simulink subsystem "AeroPropRefFranc"  (R2024b)
settings: Solver=VariableStepAuto  StartTime=0.0  StopTime=10.0  RelTol=1e-3
undefined symbols (not defined in the file or in its folder): ess, Force_b, Fprop_r, geom, H_b, Hdot_b, Moment_b, mot, mot2, mot3, mot4, Mprop_r, propel, propel2, propel3, propel4, pxf_diagram_options, SimIn, SimPar, tc, tc2, tc3, tc4
libraries: simulink x8, slpidlib x4, starslibAxisTransformations x2, libAxisTransformations x2
(part 7 of 10)

== system AeroPropRefFranc/Propulsion and Aerodynamic Forces and Moments/S-Function/Battery Model/powerplant/mot2/ctrl/dmd/parameter_selection ==
  inport-main_info_bus-1 : Inport
  select_main_info_bus : BusSelector  OutputSignals=apc_info_bus.apc_ctrl_dt2_simu,env_info_bus.env_plant_density_simu,apa_info_bus.powerplant_info_bus.ess.ctrl.ess_ctrl_pwr_max_pro_simu,apa_info_bus.powerplant_info_bus.propel2.propel2_plant_speed_simu,apa_info_bus.powerplant_info_bus.tc2.tc2_plant_spd_in_simu
  outport-apc_ctrl_dt2_simu-1 : Outport
  outport-env_plant_density_simu-2 : Outport  Port=2
  outport-ess_ctrl_pwr_max_pro_simu-3 : Outport  Port=3
  outport-propel2_plant_speed_simu-4 : Outport  Port=4
  outport-tc2_plant_spd_in_simu-5 : Outport  Port=5
  wires:
  select_main_info_bus/5 -> outport-tc2_plant_spd_in_simu-5/1  "<tc2_plant_spd_in_simu>"
  select_main_info_bus/4 -> outport-propel2_plant_speed_simu-4/1  "<propel2_plant_speed_simu>"
  select_main_info_bus/3 -> outport-ess_ctrl_pwr_max_pro_simu-3/1  "<ess_ctrl_pwr_max_pro_simu>"
  select_main_info_bus/2 -> outport-env_plant_density_simu-2/1  "<env_plant_density_simu>"
  select_main_info_bus/1 -> outport-apc_ctrl_dt2_simu-1/1  "<apc_ctrl_dt2_simu>"
  inport-main_info_bus-1/1 -> select_main_info_bus/1

== system AeroPropRefFranc/Propulsion and Aerodynamic Forces and Moments/S-Function/Battery Model/powerplant/mot2/plant/mot2_plant_map_Pelec_funTW_volt_in/electric machine filter ==
  trq : Inport
  Interval Test : simulink/Logic and Bit Operations/Interval Test  IntervalClosedRight=on  uplimit=0.02  IntervalClosedLeft=on  lowlimit=-0.02  OutDataTypeStr=boolean
  Switch : Switch  Threshold=0.5  SaturateOnIntegerOverflow=off  InputSameDT=off
  electric machine time response : TransferFcn  Denominator=[mot2.plant.init.time_response 1]
  filtered : Outport
  wires:
  electric machine time response/1 -> Switch/3
  Interval Test/1 -> Switch/2
  trq/1 -> Switch/1, Interval Test/1, electric machine time response/1
  Switch/1 -> filtered/1

== system AeroPropRefFranc/Propulsion and Aerodynamic Forces and Moments/S-Function/Battery Model/powerplant/mot2/plant/mot2_plant_map_Pelec_funTW_volt_in/max torque  ==
  cmd : Inport
  speed : Inport  Port=2
  torque : Inport  Port=3
  Abs : Abs
  Cont trq max - Prop : Subsystem  mask{x=mot2.plant.init.trq_pos_cont.idx1_spd, map=mot2.plant.init.trq_pos_cont.map}
      mask Display: image(imread('map1D.jpg','jpeg'))
  Cont trq max - Regen : Subsystem  mask{x=mot2.plant.init.trq_neg_cont.idx1_spd, map=mot2.plant.init.trq_neg_cont.map}
      mask Display: image(imread('map1D.jpg','jpeg'))
  Heat index : Subsystem
  Memory : Memory
  Peak trq max - Prop : Subsystem  mask{x=mot2.plant.init.trq_pos_max.idx1_spd, map=mot2.plant.init.trq_pos_max.map}
      mask Display: image(imread('map1D.jpg','jpeg'))
  Peak trq max - Regen : Subsystem  mask{x=mot2.plant.init.trq_neg_max.idx1_spd, map=mot2.plant.init.trq_neg_max.map}
      mask Display: image(imread('map1D.jpg','jpeg'))
  Product2 : Product  InputSameDT=on  SaturateOnIntegerOverflow=on  OutDataTypeStr=Inherit: Same as first input
  Product3 : Product  InputSameDT=on  SaturateOnIntegerOverflow=on  OutDataTypeStr=Inherit: Same as first input
  Product5 : Product  InputSameDT=on  SaturateOnIntegerOverflow=on  OutDataTypeStr=Inherit: Same as first input
  Sign : Signum
  Sum : Sum  InputSameDT=on  SaturateOnIntegerOverflow=on  OutDataTypeStr=Inherit: Same as first input
  Sum1 : Sum  Inputs=-+  InputSameDT=on  SaturateOnIntegerOverflow=on  OutDataTypeStr=Inherit: Same as first input
  Switch : Switch  InputSameDT=off
  Switch1 : Switch  InputSameDT=off
  cst : Constant
  max torque : Outport
  heat index : Outport  Port=2
  wires:
  Heat index/1(Heat index) -> heat index/1, Sum1/1, Product2/2
  cst/1 -> Sum1/2
  Product3/1 -> Sum/2
  Sum1/1 -> Product3/1
  Product2/1 -> Sum/1
  Switch1/1 -> Product3/2
  Switch/1 -> Heat index/1(cont torque), Product2/1
  Peak trq max - Regen/1(output) -> Switch1/3
  Peak trq max - Prop/1(output) -> Switch1/1
  Cont trq max - Regen/1(output) -> Switch/3
  Cont trq max - Prop/1(output) -> Switch/1
  speed/1 -> Memory/1
  cmd/1 -> Switch/2, Switch1/2
  torque/1 -> Heat index/2(torque)
  Abs/1 -> Product5/2
  Sum/1 -> Abs/1, Sign/1
  Product5/1 -> max torque/1
  Sign/1 -> Product5/1
  Memory/1 -> Peak trq max - Prop/1(input x), Peak trq max - Regen/1(input x), Cont trq max - Regen/1(input x), Cont trq max - Prop/1(input x)

== system AeroPropRefFranc/Propulsion and Aerodynamic Forces and Moments/S-Function/Battery Model/powerplant/mot2/plant/mot2_plant_map_Pelec_funTW_volt_in/non-zero division ==
  note: original idea from Phil Sharer - ANL
      | original formula: u[1]\(u[2]+eps)*(u[2]!=0)
      | changes done by Gerald ZINI (dgey) - ANL (05\02\2001)
  note: (u[2]==0) is true then returns 1, thus (u[2]+(u[2]==0)) is equal to 0+1=1
  note: if u[2] == 0, then output == 0:
  note: (u[2]!=0) is false then returns 0
  note: and finally, the expression is: (u[1] \ 1) * 0 = 0
  note: (u[2]==0) is false then returns 0, thus (u[2]+(u[2]==0)) is equal to u[2]+0=u[2]
  note: if u[2] != 0, then output == u[1]\u[2]:
  note: (u[2]!=0) is true then returns 1
  note: and finally, the expression is: (u[1] \ u[2]) * 1 = u[1] \ u[2]
  In1 : Inport
  In2 : Inport  Port=2
  Fcn : Fcn  Expr=u[1]/(u[2]+(u[2]==0))*(u[2]!=0)
  Mux : Mux  Inputs=2
  Out1 : Outport
  wires:
  Mux/1 -> Fcn/1
  In1/1 -> Mux/1
  Fcn/1 -> Out1/1
  In2/1 -> Mux/2

== system AeroPropRefFranc/Propulsion and Aerodynamic Forces and Moments/S-Function/Battery Model/powerplant/mot3/ctrl/cmd/mot3_ctrl_cmd_map_Pelec_funTW_volt_in ==
  mot_plant_spd_out_simu : Inport
  mot_ctrl_trs_trq_simu : Inport  Port=2
  mot_ctrl_cstr_trq_max_pos_simu : Inport  Port=3
  mot_ctrl_cstr_trq_max_neg_simu : Inport  Port=4
  Abs : Abs
  Abs1 : Abs
  Abs2 : Abs
  Fcn : Fcn  Expr=(u>=0) - (u<0)
  Product : Product  SaturateOnIntegerOverflow=on  OutDataTypeStr=Inherit: Same as first input
  Product1 : Product  SaturateOnIntegerOverflow=on  OutDataTypeStr=Inherit: Same as first input
  Subsystem2 : Subsystem
      mask Display: disp('divider')
  Switch : Switch  InputSameDT=off
  "[-1, 1]" : Saturate  UpperLimit=1  LowerLimit=-1
  avoid zero output : Subsystem
  mot_ctrl_cmd_simu : Outport
  wires:
  Fcn/1 -> Product1/1
  "[-1, 1]"/1 -> Product1/2
  Abs2/1 -> Switch/3
  Abs1/1 -> Switch/1
  Abs/1 -> Subsystem2/1(In1)
  mot_ctrl_trs_trq_simu/1 -> Abs/1, Product/1
  Subsystem2/1(Out1) -> "[-1, 1]"/1
  Switch/1 -> Subsystem2/2(In2)
  Product/1 -> Fcn/1, Switch/2
  mot_plant_spd_out_simu/1 -> avoid zero output/1(In1)
  mot_ctrl_cstr_trq_max_neg_simu/1 -> Abs2/1
  mot_ctrl_cstr_trq_max_pos_simu/1 -> Abs1/1
  Product1/1 -> [mot3_ctrl_cmd_simu]
  [mot3_ctrl_cmd_simu] -> mot_ctrl_cmd_simu/1  "mot_ctrl_cmd_simu"
  avoid zero output/1(Out1) -> Product/2

== system AeroPropRefFranc/Propulsion and Aerodynamic Forces and Moments/S-Function/Battery Model/powerplant/mot3/ctrl/cmd/parameter_out ==
  inport-mot3_ctrl_cmd_simu : Inport
  Toworkspace-mot3_ctrl_cmd_simu : ToWorkspace  VariableName=mot3_ctrl_cmd_simu  SampleTime=pxf_diagram_options.workspace_sample_time
      settings: Decimation=pxf_diagram_options.decimation
  create_system_info_bus : BusCreator  Inputs=1
  outport-system_info_bus : Outport
  wires:
  inport-mot3_ctrl_cmd_simu/1 -> Toworkspace-mot3_ctrl_cmd_simu/1, create_system_info_bus/1  "mot3_ctrl_cmd_simu"
  create_system_info_bus/1 -> outport-system_info_bus/1

== system AeroPropRefFranc/Propulsion and Aerodynamic Forces and Moments/S-Function/Battery Model/powerplant/mot3/ctrl/cmd/parameter_selection ==
  inport-main_info_bus-1 : Inport
  select_main_info_bus : BusSelector  OutputSignals=apa_info_bus.powerplant_info_bus.mot3.plant.mot3_plant_spd_out_simu,apa_info_bus.powerplant_info_bus.mot3.ctrl.dmd.mot3_ctrl_trs_trq_simu,apa_info_bus.powerplant_info_bus.mot3.ctrl.cstr.mot3_ctrl_cstr_trq_max_pos_simu,apa_info_bus.powerplant_info_bus.mot3.ctrl.cstr.mot3_ctrl_cstr_trq_max_neg_simu
  outport-mot3_plant_spd_out_simu-1 : Outport
  outport-mot3_ctrl_trs_trq_simu-2 : Outport  Port=2
  outport-mot3_ctrl_cstr_trq_max_pos_simu-3 : Outport  Port=3
  outport-mot3_ctrl_cstr_trq_max_neg_simu-4 : Outport  Port=4
  wires:
  select_main_info_bus/4 -> outport-mot3_ctrl_cstr_trq_max_neg_simu-4/1  "<mot3_ctrl_cstr_trq_max_neg_simu>"
  select_main_info_bus/3 -> outport-mot3_ctrl_cstr_trq_max_pos_simu-3/1  "<mot3_ctrl_cstr_trq_max_pos_simu>"
  select_main_info_bus/2 -> outport-mot3_ctrl_trs_trq_simu-2/1  "<mot3_ctrl_trs_trq_simu>"
  select_main_info_bus/1 -> outport-mot3_plant_spd_out_simu-1/1  "<mot3_plant_spd_out_simu>"
  inport-main_info_bus-1/1 -> select_main_info_bus/1

== system AeroPropRefFranc/Propulsion and Aerodynamic Forces and Moments/S-Function/Battery Model/powerplant/mot3/ctrl/cstr/mot3_ctrl_cstr_map_Pelec_funTW_volt_in ==
  mot_plant_spd_out_simu : Inport
  mot_plant_temp_coeff_simu : Inport  Port=2
  Continuous torque - Prop : Subsystem  mask{x=mot3.plant.init.trq_pos_cont.idx1_spd, map=mot3.plant.init.trq_pos_cont.map}
      mask Display: image(imread('map1D.jpg','jpeg'))
  Continuous torque _regen : Subsystem  mask{x=mot3.plant.init.trq_neg_cont.idx1_spd, map=mot3.plant.init.trq_neg_cont.map}
      mask Display: image(imread('map1D.jpg','jpeg'))
  Mux1 : Mux  Inputs=3
  Mux2 : Mux  Inputs=3
  Peak torque - Prop : Subsystem  mask{x=mot3.plant.init.trq_pos_max.idx1_spd, map=mot3.plant.init.trq_pos_max.map}
      mask Display: image(imread('map1D.jpg','jpeg'))
  Peak torque _regen : Subsystem  mask{x=mot3.plant.init.trq_neg_max.idx1_spd, map=mot3.plant.init.trq_neg_max.map}
      mask Display: image(imread('map1D.jpg','jpeg'))
  Torque1 : Fcn  Expr=u[3]*(u[2] - u[1]) + u[1]
  max torque available from meca side : Fcn  Expr=u[3]*(u[2] - u[1]) + u[1]
  mot_ctrl_cstr_trq_pk_pos_simu : Outport
  mot_ctrl_cstr_trq_max_pos_simu : Outport  Port=2
  mot_ctrl_cstr_trq_pk_neg_simu : Outport  Port=3
  mot_ctrl_cstr_trq_max_neg_simu : Outport  Port=4
  mot_ctrl_cstr_trq_cont_pos_simu : Outport  Port=5
  mot_ctrl_cstr_trq_cont_neg_simu : Outport  Port=6
  mot_ctrl_cstr_temp_coeff_simu : Outport  Port=7
  wires:
  max torque available from meca side/1 -> [mot3_ctrl_cstr_trq_max_pos_simu]
  Torque1/1 -> [mot3_ctrl_cstr_trq_max_neg_simu]
  Continuous torque - Prop/1(output) -> Mux2/2, [mot3_ctrl_cstr_trq_cont_pos_simu]
  Mux2/1 -> max torque available from meca side/1
  Continuous torque _regen/1(output) -> Mux1/2, [mot3_ctrl_cstr_trq_cont_neg_simu]
  Mux1/1 -> Torque1/1
  mot_plant_temp_coeff_simu/1 -> Mux1/3, Mux2/3, [mot3_ctrl_cstr_temp_coeff_simu]
  Peak torque - Prop/1(output) -> Mux2/1, [mot3_ctrl_cstr_trq_pk_pos_simu]
  Peak torque _regen/1(output) -> [mot3_ctrl_cstr_trq_pk_neg_simu], Mux1/1
  mot_plant_spd_out_simu/1 -> Continuous torque - Prop/1(input x), Peak torque _regen/1(input x), Continuous torque _regen/1(input x), Peak torque - Prop/1(input x)
  [mot3_ctrl_cstr_trq_pk_pos_simu] -> mot_ctrl_cstr_trq_pk_pos_simu/1  "mot_ctrl_cstr_trq_pk_pos_simu"
  [mot3_ctrl_cstr_trq_max_pos_simu] -> mot_ctrl_cstr_trq_max_pos_simu/1  "mot_ctrl_cstr_trq_max_pos_simu"
  [mot3_ctrl_cstr_trq_max_neg_simu] -> mot_ctrl_cstr_trq_max_neg_simu/1  "mot_ctrl_cstr_trq_max_neg_simu"
  [mot3_ctrl_cstr_trq_pk_neg_simu] -> mot_ctrl_cstr_trq_pk_neg_simu/1  "mot_ctrl_cstr_trq_pk_neg_simu"
  [mot3_ctrl_cstr_trq_cont_pos_simu] -> mot_ctrl_cstr_trq_cont_pos_simu/1  "mot_ctrl_cstr_trq_cont_pos_simu"
  [mot3_ctrl_cstr_trq_cont_neg_simu] -> mot_ctrl_cstr_trq_cont_neg_simu/1  "mot_ctrl_cstr_trq_cont_neg_simu"
  [mot3_ctrl_cstr_temp_coeff_simu] -> mot_ctrl_cstr_temp_coeff_simu/1  "mot_ctrl_cstr_temp_coeff_simu"

== system AeroPropRefFranc/Propulsion and Aerodynamic Forces and Moments/S-Function/Battery Model/powerplant/mot3/ctrl/cstr/parameter_out ==
  inport-mot3_ctrl_cstr_trq_pk_pos_simu : Inport
  inport-mot3_ctrl_cstr_trq_max_pos_simu : Inport  Port=2
  inport-mot3_ctrl_cstr_trq_pk_neg_simu : Inport  Port=3
  inport-mot3_ctrl_cstr_trq_max_neg_simu : Inport  Port=4
  inport-mot3_ctrl_cstr_trq_cont_pos_simu : Inport  Port=5
  inport-mot3_ctrl_cstr_trq_cont_neg_simu : Inport  Port=6
  inport-mot3_ctrl_cstr_temp_coeff_simu : Inport  Port=7
  Ground_1 : Ground
  Toworkspace-mot3_ctrl_cstr_temp_coeff_simu : ToWorkspace  VariableName=mot3_ctrl_cstr_temp_coeff_simu  SampleTime=pxf_diagram_options.workspace_sample_time
      settings: Decimation=pxf_diagram_options.decimation
  Toworkspace-mot3_ctrl_cstr_trq_cont_neg_simu : ToWorkspace  VariableName=mot3_ctrl_cstr_trq_cont_neg_simu  SampleTime=pxf_diagram_options.workspace_sample_time
      settings: Decimation=pxf_diagram_options.decimation
  Toworkspace-mot3_ctrl_cstr_trq_cont_pos_simu : ToWorkspace  VariableName=mot3_ctrl_cstr_trq_cont_pos_simu  SampleTime=pxf_diagram_options.workspace_sample_time
      settings: Decimation=pxf_diagram_options.decimation
  Toworkspace-mot3_ctrl_cstr_trq_max_neg_simu : ToWorkspace  VariableName=mot3_ctrl_cstr_trq_max_neg_simu  SampleTime=pxf_diagram_options.workspace_sample_time
      settings: Decimation=pxf_diagram_options.decimation
  Toworkspace-mot3_ctrl_cstr_trq_max_pos_simu : ToWorkspace  VariableName=mot3_ctrl_cstr_trq_max_pos_simu  SampleTime=pxf_diagram_options.workspace_sample_time
      settings: Decimation=pxf_diagram_options.decimation
  Toworkspace-mot3_ctrl_cstr_trq_pk_neg_simu : ToWorkspace  VariableName=mot3_ctrl_cstr_trq_pk_neg_simu  SampleTime=pxf_diagram_options.workspace_sample_time
      settings: Decimation=pxf_diagram_options.decimation
  Toworkspace-mot3_ctrl_cstr_trq_pk_pos_simu : ToWorkspace  VariableName=mot3_ctrl_cstr_trq_pk_pos_simu  SampleTime=pxf_diagram_options.workspace_sample_time
      settings: Decimation=pxf_diagram_options.decimation
  create_system_info_bus : BusCreator  Inputs=2
  outport-system_info_bus : Outport
  outport-cstr_bus : Outport  Port=2
  wires:
  Ground_1/1 -> outport-cstr_bus/1
  inport-mot3_ctrl_cstr_temp_coeff_simu/1 -> Toworkspace-mot3_ctrl_cstr_temp_coeff_simu/1
  inport-mot3_ctrl_cstr_trq_cont_neg_simu/1 -> Toworkspace-mot3_ctrl_cstr_trq_cont_neg_simu/1
  inport-mot3_ctrl_cstr_trq_cont_pos_simu/1 -> Toworkspace-mot3_ctrl_cstr_trq_cont_pos_simu/1
  inport-mot3_ctrl_cstr_trq_max_neg_simu/1 -> Toworkspace-mot3_ctrl_cstr_trq_max_neg_simu/1, create_system_info_bus/2  "mot3_ctrl_cstr_trq_max_neg_simu"
  inport-mot3_ctrl_cstr_trq_pk_neg_simu/1 -> Toworkspace-mot3_ctrl_cstr_trq_pk_neg_simu/1
  inport-mot3_ctrl_cstr_trq_max_pos_simu/1 -> Toworkspace-mot3_ctrl_cstr_trq_max_pos_simu/1, create_system_info_bus/1  "mot3_ctrl_cstr_trq_max_pos_simu"
  inport-mot3_ctrl_cstr_trq_pk_pos_simu/1 -> Toworkspace-mot3_ctrl_cstr_trq_pk_pos_simu/1
  create_system_info_bus/1 -> outport-system_info_bus/1

== system AeroPropRefFranc/Propulsion and Aerodynamic Forces and Moments/S-Function/Battery Model/powerplant/mot3/ctrl/cstr/parameter_selection ==
  inport-main_info_bus-1 : Inport
  select_main_info_bus : BusSelector  OutputSignals=apa_info_bus.powerplant_info_bus.mot3.plant.mot3_plant_spd_out_simu,apa_info_bus.powerplant_info_bus.mot3.plant.mot3_plant_temp_coeff_simu
  outport-mot3_plant_spd_out_simu-1 : Outport
  outport-mot3_plant_temp_coeff_simu-2 : Outport  Port=2
  wires:
  select_main_info_bus/2 -> outport-mot3_plant_temp_coeff_simu-2/1  "<mot3_plant_temp_coeff_simu>"
  select_main_info_bus/1 -> outport-mot3_plant_spd_out_simu-1/1  "<mot3_plant_spd_out_simu>"
  inport-main_info_bus-1/1 -> select_main_info_bus/1

== system AeroPropRefFranc/Propulsion and Aerodynamic Forces and Moments/S-Function/Battery Model/powerplant/mot3/ctrl/dmd/mot3_ctrl_dmd_uas ==
  apc_ctrl_dt_simu : Inport
  env_plant_density_simu : Inport  Port=2
  ess_ctrl_pwr_max_pro_simu : Inport  Port=3
  propel_plant_speed_simu : Inport  Port=4
  tc_plant_spd_in_simu : Inport  Port=5
  1\2pi1 : Gain  Gain=2*pi/mot3.tc.plant.init.ratio
  Constant : Constant  Value=mot3.propel.plant.init.Pmax
  Constant2 : Constant  Value=mot3.propel.init.CPpoly
  Constant3 : Constant  Value=0.01
  Constant8 : Constant  Value=mot3.propel.plant.init.propD
  Determine_Required_Motor_RPS : Subsystem
  Gain : Gain  Gain=1/2/pi
  Gain1 : Gain  Gain=1/2/pi
  PID Controller : slpidlib/PID Controller  Controller=PID  Form=Parallel  TimeDomain=Continuous-time  UseExternalTs=off  SampleTime=-1  IntegratorMethod=Forward Euler  FilterMethod=Forward Euler  ControllerParametersSource=internal  P=mot3.ctrl.init.P  I=mot3.ctrl.init.I  UseKiTs=off  D=mot3.ctrl.init.D  UseExternalDerivativeSource=off  N=100  UseFilter=on  TunerSelectOption=Transfer Function Based (PID Tuner App)  InitialConditionSource=internal  InitialConditionForIntegrator=0  InitialConditionForFilter=0  DifferentiatorICPrevScaledInput=0  ExternalReset=none  TrackingMode=off  Kt=1  LimitOutput=off  SatLimitsSource=internal  UpperSaturationLimit=inf  LowerSaturationLimit=-inf  LinearizeAsGain=on  AntiWindupMode=none  Kb=1  LimitIntegrator=off  UpperIntegratorSaturationLimit=inf  LowerIntegratorSaturationLimit=-inf  POutMin=[]  POutMax=[]  IOutMin=[]  IOutMax=[]  DOutMin=[]  DOutMax=[]  NOutMin=[]  NOutMax=[]  SumOutMin=[]  SumOutMax=[]  SaturationOutMin=[]  SaturationOutMax=[]  PParamMin=[]  PParamMax=[]  IParamMin=[]  IParamMax=[]  DParamMin=[]  DParamMax=[]  NParamMin=[]  NParamMax=[]  KbParamMin=[]  KbParamMax=[]  KtParamMin=[]  KtParamMax=[]  KbOutMin=[]  KbOutMax=[]  KtOutMin=[]  KtOutMax=[]  IntegratorOutMin=[]  IntegratorOutMax=[]  FilterOutMin=[]  FilterOutMax=[]  SumI1OutMin=[]  SumI1OutMax=[]  SumI2OutMin=[]  SumI2OutMax=[]  SumI3OutMin=[]  SumI3OutMax=[]  SumI4OutMin=[]  SumI4OutMax=[]  SumDOutMin=[]  SumDOutMax=[]  DifferentiatorOutMin=[]  DifferentiatorOutMax=[]  FilterDiffOutCoefMin=[]  FilterDiffOutCoefMax=[]  ReciprocalOutMin=[]  ReciprocalOutMax=[]  SumDenOutMin=[]  SumDenOutMax=[]  SumNumOutMin=[]  SumNumOutMax=[]  DivideOutMin=[]  DivideOutMax=[]  UdiffTsProdOutMin=[]  UdiffTsProdOutMax=[]  NTsProdOutMin=[]  NTsProdOutMax=[]  UintegralTsProdOutMin=[]  UintegralTsProdOutMax=[]  UngainTsProdOutMin=[]  UngainTsProdOutMax=[]  ClampingZeroOutDataTypeStr=Inherit: Inherit via back propagation  ClampingZeroOutMin=[]  ClampingZeroOutMax=[]  FilterDenConstantOutDataTypeStr=Inherit: Inherit via back propagation  FilterDenConstantOutMin=[]  FilterDenConstantOutMax=[]  PCopyOutDataTypeStr=Inherit: Inherit via back propagation  PCopyOutMin=[]  PCopyOutMax=[]  NCopyOutDataTypeStr=Inherit: Inherit via back propagation  NCopyOutMin=[]  NCopyOutMax=[]  IntegratorContinuousStateAttributes=''  IntegratorStateMustResolveToSignalObject=off  IntegratorRTWStateStorageClass=Auto  FilterContinuousStateAttributes=''  FilterStateMustResolveToSignalObject=off  FilterRTWStateStorageClass=Auto  ParallelPVariant=InternalParameters  IdealPVariant=Disabled  IVariant=InternalParameters  DVariant=InternalParameters  IntegratorVariant=Continuous  SatVariant=Disabled  AWVariant=Passthrough  PCopyVariant=Disabled  TRVariant=Disabled  FdbkBlocksVariant=Forward  IdealPFdbkVariant=Disabled  SatFdbkVariant=Disabled  DerivativeFilterVariant=ContFilter  NVariant=InternalParameters  NCopyVariant=Disabled  FilterICVariant=InternalICsFilter  IntegratorICVariant=InternalICs  ExternalResetVariant=Disabled  TRSumVariant=Passthrough  SumFdbkVariant=Disabled  SumVariant=Sum_PID  TsampFilterVariant=InternalTs  TsampNgainVariant=Passthrough  TsampIntegralVariant=Disabled_SignalSpec  ExternalSaturationOutDataTypeStr=Inherit: Same as second input  DerivativeSourceVariant=ErrorSignal  PreIntVariant=InternalPreInt
  Product2 : Product  RndMeth=Zero
  Product3 : Product
  Product4 : Product  Inputs=*/  RndMeth=Zero
  Saturation_Dynamic : simulink/Discontinuities/Saturation Dynamic  OutMin=[]  OutMax=[]  OutDataTypeStr=Inherit: Same as second input  OutDataType=fixdt(1, 16)  OutScaling=2^-10  DoSatur=off
  Sum2 : Sum  Inputs=+-|
  Sum3 : Sum  Inputs=|++
  mot_propel_plant_init_eff_map : Subsystem  mask{x=mot3.propel.plant.init.CP_CT_map(:,1)/60, map=mot3.propel.plant.init.CP_CT_map(:,4)}
  mot_ctrl_trs_trq_simu : Outport  VectorParamsAs1DForOutWhenUnconnected=off
  mot_ctrl_ratedpwr_simu : Outport  Port=2
  wires:
  Product2/1 -> Product3/1
  mot_propel_plant_init_eff_map/1(output) -> Product3/2
  Constant/1 -> mot_ctrl_ratedpwr_simu/1, Product2/1  "mot_ctrl_ratedpwr_simu"
  Constant3/1 -> Saturation_Dynamic/3
  tc_plant_spd_in_simu/1 -> Gain/1
  Saturation_Dynamic/1 -> Determine_Required_Motor_RPS/3(P), Product4/1
  Product3/1 -> Saturation_Dynamic/2
  Gain/1 -> Sum2/2  "actual"
  Product4/1 -> Sum3/1  "required"
  PID Controller/1 -> Sum3/2
  Sum3/1 -> mot_ctrl_trs_trq_simu/1  "mot_ctrl_trs_trq_simu"
  1\2pi1/1 -> Product4/2
  Sum2/1 -> PID Controller/1
  apc_ctrl_dt_simu/1 -> Product2/2
  ess_ctrl_pwr_max_pro_simu/1 -> Saturation_Dynamic/1
  propel_plant_speed_simu/1 -> Gain1/1
  Determine_Required_Motor_RPS/1(RPS_req) -> Sum2/1, 1\2pi1/1
  Constant8/1 -> Determine_Required_Motor_RPS/1(Prop_D)
  env_plant_density_simu/1 -> Determine_Required_Motor_RPS/2(rho)
  Constant2/1 -> Determine_Required_Motor_RPS/4(CPpoly)
  Gain1/1 -> mot_propel_plant_init_eff_map/1(input x)

== system AeroPropRefFranc/Propulsion and Aerodynamic Forces and Moments/S-Function/Battery Model/powerplant/mot3/ctrl/dmd/parameter_out ==
  inport-mot3_ctrl_trs_trq_simu : Inport
  inport-mot3_ctrl_ratedpwr_simu : Inport  Port=2
  Ground_1 : Ground
  Toworkspace-mot3_ctrl_ratedpwr_simu : ToWorkspace  VariableName=mot3_ctrl_ratedpwr_simu  SampleTime=pxf_diagram_options.workspace_sample_time
      settings: Decimation=pxf_diagram_options.decimation
  Toworkspace-mot3_ctrl_trs_trq_simu : ToWorkspace  VariableName=mot3_ctrl_trs_trq_simu  SampleTime=pxf_diagram_options.workspace_sample_time
      settings: Decimation=pxf_diagram_options.decimation
  create_system_info_bus : BusCreator  Inputs=1
  outport-system_info_bus : Outport
  outport-dmd_bus : Outport  Port=2
  wires:
  Ground_1/1 -> outport-dmd_bus/1
  inport-mot3_ctrl_ratedpwr_simu/1 -> Toworkspace-mot3_ctrl_ratedpwr_simu/1
  inport-mot3_ctrl_trs_trq_simu/1 -> Toworkspace-mot3_ctrl_trs_trq_simu/1, create_system_info_bus/1  "mot3_ctrl_trs_trq_simu"
  create_system_info_bus/1 -> outport-system_info_bus/1

== system AeroPropRefFranc/Propulsion and Aerodynamic Forces and Moments/S-Function/Battery Model/powerplant/mot3/ctrl/dmd/parameter_selection ==
  inport-main_info_bus-1 : Inport
  select_main_info_bus : BusSelector  OutputSignals=apc_info_bus.apc_ctrl_dt3_simu,env_info_bus.env_plant_density_simu,apa_info_bus.powerplant_info_bus.ess.ctrl.ess_ctrl_pwr_max_pro_simu,apa_info_bus.powerplant_info_bus.propel3.propel3_plant_speed_simu,apa_info_bus.powerplant_info_bus.tc3.tc3_plant_spd_in_simu
  outport-apc_ctrl_dt3_simu-1 : Outport
  outport-env_plant_density_simu-2 : Outport  Port=2
  outport-ess_ctrl_pwr_max_pro_simu-3 : Outport  Port=3
  outport-propel3_plant_speed_simu-4 : Outport  Port=4
  outport-tc3_plant_spd_in_simu-5 : Outport  Port=5
  wires:
  select_main_info_bus/5 -> outport-tc3_plant_spd_in_simu-5/1  "<tc3_plant_spd_in_simu>"
  select_main_info_bus/4 -> outport-propel3_plant_speed_simu-4/1  "<propel3_plant_speed_simu>"
  select_main_info_bus/3 -> outport-ess_ctrl_pwr_max_pro_simu-3/1  "<ess_ctrl_pwr_max_pro_simu>"
  select_main_info_bus/2 -> outport-env_plant_density_simu-2/1  "<env_plant_density_simu>"
  select_main_info_bus/1 -> outport-apc_ctrl_dt3_simu-1/1  "<apc_ctrl_dt3_simu>"
  inport-main_info_bus-1/1 -> select_main_info_bus/1

== system AeroPropRefFranc/Propulsion and Aerodynamic Forces and Moments/S-Function/Battery Model/powerplant/mot3/plant/mot3_plant_map_Pelec_funTW_volt_in/electric machine filter ==
  trq : Inport
  Interval Test : simulink/Logic and Bit Operations/Interval Test  IntervalClosedRight=on  uplimit=0.02  IntervalClosedLeft=on  lowlimit=-0.02  OutDataTypeStr=boolean
  Switch : Switch  Threshold=0.5  SaturateOnIntegerOverflow=off  InputSameDT=off
  electric machine time response : TransferFcn  Denominator=[mot3.plant.init.time_response 1]
  filtered : Outport
  wires:
  electric machine time response/1 -> Switch/3
  Interval Test/1 -> Switch/2
  trq/1 -> Switch/1, Interval Test/1, electric machine time response/1
  Switch/1 -> filtered/1

== system AeroPropRefFranc/Propulsion and Aerodynamic Forces and Moments/S-Function/Battery Model/powerplant/mot3/plant/mot3_plant_map_Pelec_funTW_volt_in/max torque  ==
  cmd : Inport
  speed : Inport  Port=2
  torque : Inport  Port=3
  Abs : Abs
  Cont trq max - Prop : Subsystem  mask{x=mot3.plant.init.trq_pos_cont.idx1_spd, map=mot3.plant.init.trq_pos_cont.map}
      mask Display: image(imread('map1D.jpg','jpeg'))
  Cont trq max - Regen : Subsystem  mask{x=mot3.plant.init.trq_neg_cont.idx1_spd, map=mot3.plant.init.trq_neg_cont.map}
      mask Display: image(imread('map1D.jpg','jpeg'))
  Heat index : Subsystem
  Memory : Memory
  Peak trq max - Prop : Subsystem  mask{x=mot3.plant.init.trq_pos_max.idx1_spd, map=mot3.plant.init.trq_pos_max.map}
      mask Display: image(imread('map1D.jpg','jpeg'))
  Peak trq max - Regen : Subsystem  mask{x=mot3.plant.init.trq_neg_max.idx1_spd, map=mot3.plant.init.trq_neg_max.map}
      mask Display: image(imread('map1D.jpg','jpeg'))
  Product2 : Product  InputSameDT=on  SaturateOnIntegerOverflow=on  OutDataTypeStr=Inherit: Same as first input
  Product3 : Product  InputSameDT=on  SaturateOnIntegerOverflow=on  OutDataTypeStr=Inherit: Same as first input
  Product5 : Product  InputSameDT=on  SaturateOnIntegerOverflow=on  OutDataTypeStr=Inherit: Same as first input
  Sign : Signum
  Sum : Sum  InputSameDT=on  SaturateOnIntegerOverflow=on  OutDataTypeStr=Inherit: Same as first input
  Sum1 : Sum  Inputs=-+  InputSameDT=on  SaturateOnIntegerOverflow=on  OutDataTypeStr=Inherit: Same as first input
  Switch : Switch  InputSameDT=off
  Switch1 : Switch  InputSameDT=off
  cst : Constant
  max torque : Outport
  heat index : Outport  Port=2
  wires:
  Heat index/1(Heat index) -> heat index/1, Sum1/1, Product2/2
  cst/1 -> Sum1/2
  Product3/1 -> Sum/2
  Sum1/1 -> Product3/1
  Product2/1 -> Sum/1
  Switch1/1 -> Product3/2
  Switch/1 -> Heat index/1(cont torque), Product2/1
  Peak trq max - Regen/1(output) -> Switch1/3
  Peak trq max - Prop/1(output) -> Switch1/1
  Cont trq max - Regen/1(output) -> Switch/3
  Cont trq max - Prop/1(output) -> Switch/1
  speed/1 -> Memory/1
  cmd/1 -> Switch/2, Switch1/2
  torque/1 -> Heat index/2(torque)
  Abs/1 -> Product5/2
  Sum/1 -> Abs/1, Sign/1
  Product5/1 -> max torque/1
  Sign/1 -> Product5/1
  Memory/1 -> Peak trq max - Prop/1(input x), Peak trq max - Regen/1(input x), Cont trq max - Regen/1(input x), Cont trq max - Prop/1(input x)

== system AeroPropRefFranc/Propulsion and Aerodynamic Forces and Moments/S-Function/Battery Model/powerplant/mot3/plant/mot3_plant_map_Pelec_funTW_volt_in/non-zero division ==
  note: original idea from Phil Sharer - ANL
      | original formula: u[1]\(u[2]+eps)*(u[2]!=0)
      | changes done by Gerald ZINI (dgey) - ANL (05\02\2001)
  note: (u[2]==0) is true then returns 1, thus (u[2]+(u[2]==0)) is equal to 0+1=1
  note: if u[2] == 0, then output == 0:
  note: (u[2]!=0) is false then returns 0
  note: and finally, the expression is: (u[1] \ 1) * 0 = 0
  note: (u[2]==0) is false then returns 0, thus (u[2]+(u[2]==0)) is equal to u[2]+0=u[2]
  note: if u[2] != 0, then output == u[1]\u[2]:
  note: (u[2]!=0) is true then returns 1
  note: and finally, the expression is: (u[1] \ u[2]) * 1 = u[1] \ u[2]
  In1 : Inport
  In2 : Inport  Port=2
  Fcn : Fcn  Expr=u[1]/(u[2]+(u[2]==0))*(u[2]!=0)
  Mux : Mux  Inputs=2
  Out1 : Outport
  wires:
  Mux/1 -> Fcn/1
  In1/1 -> Mux/1
  Fcn/1 -> Out1/1
  In2/1 -> Mux/2

== system AeroPropRefFranc/Propulsion and Aerodynamic Forces and Moments/S-Function/Battery Model/powerplant/mot4/ctrl/cmd/mot4_ctrl_cmd_map_Pelec_funTW_volt_in ==
  mot_plant_spd_out_simu : Inport
  mot_ctrl_trs_trq_simu : Inport  Port=2
  mot_ctrl_cstr_trq_max_pos_simu : Inport  Port=3
  mot_ctrl_cstr_trq_max_neg_simu : Inport  Port=4
  Abs : Abs
  Abs1 : Abs
  Abs2 : Abs
  Fcn : Fcn  Expr=(u>=0) - (u<0)
  Product : Product  SaturateOnIntegerOverflow=on  OutDataTypeStr=Inherit: Same as first input
  Product1 : Product  SaturateOnIntegerOverflow=on  OutDataTypeStr=Inherit: Same as first input
  Subsystem2 : Subsystem
      mask Display: disp('divider')
  Switch : Switch  InputSameDT=off
  "[-1, 1]" : Saturate  UpperLimit=1  LowerLimit=-1
  avoid zero output : Subsystem
  mot_ctrl_cmd_simu : Outport
  wires:
  Fcn/1 -> Product1/1
  "[-1, 1]"/1 -> Product1/2
  Abs2/1 -> Switch/3
  Abs1/1 -> Switch/1
  Abs/1 -> Subsystem2/1(In1)
  mot_ctrl_trs_trq_simu/1 -> Abs/1, Product/1
  Subsystem2/1(Out1) -> "[-1, 1]"/1
  Switch/1 -> Subsystem2/2(In2)
  Product/1 -> Fcn/1, Switch/2
  mot_plant_spd_out_simu/1 -> avoid zero output/1(In1)
  mot_ctrl_cstr_trq_max_neg_simu/1 -> Abs2/1
  mot_ctrl_cstr_trq_max_pos_simu/1 -> Abs1/1
  Product1/1 -> [mot4_ctrl_cmd_simu]
  [mot4_ctrl_cmd_simu] -> mot_ctrl_cmd_simu/1  "mot_ctrl_cmd_simu"
  avoid zero output/1(Out1) -> Product/2

== system AeroPropRefFranc/Propulsion and Aerodynamic Forces and Moments/S-Function/Battery Model/powerplant/mot4/ctrl/cmd/parameter_out ==
  inport-mot4_ctrl_cmd_simu : Inport
  Toworkspace-mot4_ctrl_cmd_simu : ToWorkspace  VariableName=mot4_ctrl_cmd_simu  SampleTime=pxf_diagram_options.workspace_sample_time
      settings: Decimation=pxf_diagram_options.decimation
  create_system_info_bus : BusCreator  Inputs=1
  outport-system_info_bus : Outport
  wires:
  inport-mot4_ctrl_cmd_simu/1 -> Toworkspace-mot4_ctrl_cmd_simu/1, create_system_info_bus/1  "mot4_ctrl_cmd_simu"
  create_system_info_bus/1 -> outport-system_info_bus/1

== system AeroPropRefFranc/Propulsion and Aerodynamic Forces and Moments/S-Function/Battery Model/powerplant/mot4/ctrl/cmd/parameter_selection ==
  inport-main_info_bus-1 : Inport
  select_main_info_bus : BusSelector  OutputSignals=apa_info_bus.powerplant_info_bus.mot4.plant.mot4_plant_spd_out_simu,apa_info_bus.powerplant_info_bus.mot4.ctrl.dmd.mot4_ctrl_trs_trq_simu,apa_info_bus.powerplant_info_bus.mot4.ctrl.cstr.mot4_ctrl_cstr_trq_max_pos_simu,apa_info_bus.powerplant_info_bus.mot4.ctrl.cstr.mot4_ctrl_cstr_trq_max_neg_simu
  outport-mot4_plant_spd_out_simu-1 : Outport
  outport-mot4_ctrl_trs_trq_simu-2 : Outport  Port=2
  outport-mot4_ctrl_cstr_trq_max_pos_simu-3 : Outport  Port=3
  outport-mot4_ctrl_cstr_trq_max_neg_simu-4 : Outport  Port=4
  wires:
  select_main_info_bus/4 -> outport-mot4_ctrl_cstr_trq_max_neg_simu-4/1  "<mot4_ctrl_cstr_trq_max_neg_simu>"
  select_main_info_bus/3 -> outport-mot4_ctrl_cstr_trq_max_pos_simu-3/1  "<mot4_ctrl_cstr_trq_max_pos_simu>"
  select_main_info_bus/2 -> outport-mot4_ctrl_trs_trq_simu-2/1  "<mot4_ctrl_trs_trq_simu>"
  select_main_info_bus/1 -> outport-mot4_plant_spd_out_simu-1/1  "<mot4_plant_spd_out_simu>"
  inport-main_info_bus-1/1 -> select_main_info_bus/1

== system AeroPropRefFranc/Propulsion and Aerodynamic Forces and Moments/S-Function/Battery Model/powerplant/mot4/ctrl/cstr/mot4_ctrl_cstr_map_Pelec_funTW_volt_in ==
  mot_plant_spd_out_simu : Inport
  mot_plant_temp_coeff_simu : Inport  Port=2
  Continuous torque - Prop : Subsystem  mask{x=mot4.plant.init.trq_pos_cont.idx1_spd, map=mot4.plant.init.trq_pos_cont.map}
      mask Display: image(imread('map1D.jpg','jpeg'))
  Continuous torque _regen : Subsystem  mask{x=mot4.plant.init.trq_neg_cont.idx1_spd, map=mot4.plant.init.trq_neg_cont.map}
      mask Display: image(imread('map1D.jpg','jpeg'))
  Mux1 : Mux  Inputs=3
  Mux2 : Mux  Inputs=3
  Peak torque - Prop : Subsystem  mask{x=mot4.plant.init.trq_pos_max.idx1_spd, map=mot4.plant.init.trq_pos_max.map}
      mask Display: image(imread('map1D.jpg','jpeg'))
  Peak torque _regen : Subsystem  mask{x=mot4.plant.init.trq_neg_max.idx1_spd, map=mot4.plant.init.trq_neg_max.map}
      mask Display: image(imread('map1D.jpg','jpeg'))
  Torque1 : Fcn  Expr=u[3]*(u[2] - u[1]) + u[1]
  max torque available from meca side : Fcn  Expr=u[3]*(u[2] - u[1]) + u[1]
  mot_ctrl_cstr_trq_pk_pos_simu : Outport
  mot_ctrl_cstr_trq_max_pos_simu : Outport  Port=2
  mot_ctrl_cstr_trq_pk_neg_simu : Outport  Port=3
  mot_ctrl_cstr_trq_max_neg_simu : Outport  Port=4
  mot_ctrl_cstr_trq_cont_pos_simu : Outport  Port=5
  mot_ctrl_cstr_trq_cont_neg_simu : Outport  Port=6
  mot_ctrl_cstr_temp_coeff_simu : Outport  Port=7
  wires:
  max torque available from meca side/1 -> [mot4_ctrl_cstr_trq_max_pos_simu]
  Torque1/1 -> [mot4_ctrl_cstr_trq_max_neg_simu]
  Continuous torque - Prop/1(output) -> Mux2/2, [mot4_ctrl_cstr_trq_cont_pos_simu]
  Mux2/1 -> max torque available from meca side/1
  Continuous torque _regen/1(output) -> Mux1/2, [mot4_ctrl_cstr_trq_cont_neg_simu]
  Mux1/1 -> Torque1/1
  mot_plant_temp_coeff_simu/1 -> Mux1/3, Mux2/3, [mot4_ctrl_cstr_temp_coeff_simu]
  Peak torque - Prop/1(output) -> Mux2/1, [mot4_ctrl_cstr_trq_pk_pos_simu]
  Peak torque _regen/1(output) -> [mot4_ctrl_cstr_trq_pk_neg_simu], Mux1/1
  mot_plant_spd_out_simu/1 -> Continuous torque - Prop/1(input x), Peak torque _regen/1(input x), Continuous torque _regen/1(input x), Peak torque - Prop/1(input x)
  [mot4_ctrl_cstr_trq_pk_pos_simu] -> mot_ctrl_cstr_trq_pk_pos_simu/1  "mot_ctrl_cstr_trq_pk_pos_simu"
  [mot4_ctrl_cstr_trq_max_pos_simu] -> mot_ctrl_cstr_trq_max_pos_simu/1  "mot_ctrl_cstr_trq_max_pos_simu"
  [mot4_ctrl_cstr_trq_max_neg_simu] -> mot_ctrl_cstr_trq_max_neg_simu/1  "mot_ctrl_cstr_trq_max_neg_simu"
  [mot4_ctrl_cstr_trq_pk_neg_simu] -> mot_ctrl_cstr_trq_pk_neg_simu/1  "mot_ctrl_cstr_trq_pk_neg_simu"
  [mot4_ctrl_cstr_trq_cont_pos_simu] -> mot_ctrl_cstr_trq_cont_pos_simu/1  "mot_ctrl_cstr_trq_cont_pos_simu"
  [mot4_ctrl_cstr_trq_cont_neg_simu] -> mot_ctrl_cstr_trq_cont_neg_simu/1  "mot_ctrl_cstr_trq_cont_neg_simu"
  [mot4_ctrl_cstr_temp_coeff_simu] -> mot_ctrl_cstr_temp_coeff_simu/1  "mot_ctrl_cstr_temp_coeff_simu"

== system AeroPropRefFranc/Propulsion and Aerodynamic Forces and Moments/S-Function/Battery Model/powerplant/mot4/ctrl/cstr/parameter_out ==
  inport-mot4_ctrl_cstr_trq_pk_pos_simu : Inport
  inport-mot4_ctrl_cstr_trq_max_pos_simu : Inport  Port=2
  inport-mot4_ctrl_cstr_trq_pk_neg_simu : Inport  Port=3
  inport-mot4_ctrl_cstr_trq_max_neg_simu : Inport  Port=4
  inport-mot4_ctrl_cstr_trq_cont_pos_simu : Inport  Port=5
  inport-mot4_ctrl_cstr_trq_cont_neg_simu : Inport  Port=6
  inport-mot4_ctrl_cstr_temp_coeff_simu : Inport  Port=7
  Ground_1 : Ground
  Toworkspace-mot4_ctrl_cstr_temp_coeff_simu : ToWorkspace  VariableName=mot4_ctrl_cstr_temp_coeff_simu  SampleTime=pxf_diagram_options.workspace_sample_time
      settings: Decimation=pxf_diagram_options.decimation
  Toworkspace-mot4_ctrl_cstr_trq_cont_neg_simu : ToWorkspace  VariableName=mot4_ctrl_cstr_trq_cont_neg_simu  SampleTime=pxf_diagram_options.workspace_sample_time
      settings: Decimation=pxf_diagram_options.decimation
  Toworkspace-mot4_ctrl_cstr_trq_cont_pos_simu : ToWorkspace  VariableName=mot4_ctrl_cstr_trq_cont_pos_simu  SampleTime=pxf_diagram_options.workspace_sample_time
      settings: Decimation=pxf_diagram_options.decimation
  Toworkspace-mot4_ctrl_cstr_trq_max_neg_simu : ToWorkspace  VariableName=mot4_ctrl_cstr_trq_max_neg_simu  SampleTime=pxf_diagram_options.workspace_sample_time
      settings: Decimation=pxf_diagram_options.decimation
  Toworkspace-mot4_ctrl_cstr_trq_max_pos_simu : ToWorkspace  VariableName=mot4_ctrl_cstr_trq_max_pos_simu  SampleTime=pxf_diagram_options.workspace_sample_time
      settings: Decimation=pxf_diagram_options.decimation
  Toworkspace-mot4_ctrl_cstr_trq_pk_neg_simu : ToWorkspace  VariableName=mot4_ctrl_cstr_trq_pk_neg_simu  SampleTime=pxf_diagram_options.workspace_sample_time
      settings: Decimation=pxf_diagram_options.decimation
  Toworkspace-mot4_ctrl_cstr_trq_pk_pos_simu : ToWorkspace  VariableName=mot4_ctrl_cstr_trq_pk_pos_simu  SampleTime=pxf_diagram_options.workspace_sample_time
      settings: Decimation=pxf_diagram_options.decimation
  create_system_info_bus : BusCreator  Inputs=2
  outport-system_info_bus : Outport
  outport-cstr_bus : Outport  Port=2
  wires:
  Ground_1/1 -> outport-cstr_bus/1
  inport-mot4_ctrl_cstr_temp_coeff_simu/1 -> Toworkspace-mot4_ctrl_cstr_temp_coeff_simu/1
  inport-mot4_ctrl_cstr_trq_cont_neg_simu/1 -> Toworkspace-mot4_ctrl_cstr_trq_cont_neg_simu/1
  inport-mot4_ctrl_cstr_trq_cont_pos_simu/1 -> Toworkspace-mot4_ctrl_cstr_trq_cont_pos_simu/1
  inport-mot4_ctrl_cstr_trq_max_neg_simu/1 -> Toworkspace-mot4_ctrl_cstr_trq_max_neg_simu/1, create_system_info_bus/2  "mot4_ctrl_cstr_trq_max_neg_simu"
  inport-mot4_ctrl_cstr_trq_pk_neg_simu/1 -> Toworkspace-mot4_ctrl_cstr_trq_pk_neg_simu/1
  inport-mot4_ctrl_cstr_trq_max_pos_simu/1 -> Toworkspace-mot4_ctrl_cstr_trq_max_pos_simu/1, create_system_info_bus/1  "mot4_ctrl_cstr_trq_max_pos_simu"
  inport-mot4_ctrl_cstr_trq_pk_pos_simu/1 -> Toworkspace-mot4_ctrl_cstr_trq_pk_pos_simu/1
  create_system_info_bus/1 -> outport-system_info_bus/1

== system AeroPropRefFranc/Propulsion and Aerodynamic Forces and Moments/S-Function/Battery Model/powerplant/mot4/ctrl/cstr/parameter_selection ==
  inport-main_info_bus-1 : Inport
  select_main_info_bus : BusSelector  OutputSignals=apa_info_bus.powerplant_info_bus.mot4.plant.mot4_plant_spd_out_simu,apa_info_bus.powerplant_info_bus.mot4.plant.mot4_plant_temp_coeff_simu
  outport-mot4_plant_spd_out_simu-1 : Outport
  outport-mot4_plant_temp_coeff_simu-2 : Outport  Port=2
  wires:
  select_main_info_bus/2 -> outport-mot4_plant_temp_coeff_simu-2/1  "<mot4_plant_temp_coeff_simu>"
  select_main_info_bus/1 -> outport-mot4_plant_spd_out_simu-1/1  "<mot4_plant_spd_out_simu>"
  inport-main_info_bus-1/1 -> select_main_info_bus/1

== system AeroPropRefFranc/Propulsion and Aerodynamic Forces and Moments/S-Function/Battery Model/powerplant/mot4/ctrl/dmd/mot4_ctrl_dmd_uas ==
  apc_ctrl_dt_simu : Inport
  env_plant_density_simu : Inport  Port=2
  ess_ctrl_pwr_max_pro_simu : Inport  Port=3
  propel_plant_speed_simu : Inport  Port=4
  tc_plant_spd_in_simu : Inport  Port=5
  1\2pi1 : Gain  Gain=2*pi/mot4.tc.plant.init.ratio
  Constant : Constant  Value=mot4.propel.plant.init.Pmax
  Constant2 : Constant  Value=mot4.propel.init.CPpoly
  Constant3 : Constant  Value=0.01
  Constant8 : Constant  Value=mot4.propel.plant.init.propD
  Determine_Required_Motor_RPS : Subsystem
  Gain : Gain  Gain=1/2/pi
  Gain1 : Gain  Gain=1/2/pi
  PID Controller : slpidlib/PID Controller  Controller=PID  Form=Parallel  TimeDomain=Continuous-time  UseExternalTs=off  SampleTime=-1  IntegratorMethod=Forward Euler  FilterMethod=Forward Euler  ControllerParametersSource=internal  P=mot4.ctrl.init.P  I=mot4.ctrl.init.I  UseKiTs=off  D=mot4.ctrl.init.D  UseExternalDerivativeSource=off  N=100  UseFilter=on  TunerSelectOption=Transfer Function Based (PID Tuner App)  InitialConditionSource=internal  InitialConditionForIntegrator=0  InitialConditionForFilter=0  DifferentiatorICPrevScaledInput=0  ExternalReset=none  TrackingMode=off  Kt=1  LimitOutput=off  SatLimitsSource=internal  UpperSaturationLimit=inf  LowerSaturationLimit=-inf  LinearizeAsGain=on  AntiWindupMode=none  Kb=1  LimitIntegrator=off  UpperIntegratorSaturationLimit=inf  LowerIntegratorSaturationLimit=-inf  POutMin=[]  POutMax=[]  IOutMin=[]  IOutMax=[]  DOutMin=[]  DOutMax=[]  NOutMin=[]  NOutMax=[]  SumOutMin=[]  SumOutMax=[]  SaturationOutMin=[]  SaturationOutMax=[]  PParamMin=[]  PParamMax=[]  IParamMin=[]  IParamMax=[]  DParamMin=[]  DParamMax=[]  NParamMin=[]  NParamMax=[]  KbParamMin=[]  KbParamMax=[]  KtParamMin=[]  KtParamMax=[]  KbOutMin=[]  KbOutMax=[]  KtOutMin=[]  KtOutMax=[]  IntegratorOutMin=[]  IntegratorOutMax=[]  FilterOutMin=[]  FilterOutMax=[]  SumI1OutMin=[]  SumI1OutMax=[]  SumI2OutMin=[]  SumI2OutMax=[]  SumI3OutMin=[]  SumI3OutMax=[]  SumI4OutMin=[]  SumI4OutMax=[]  SumDOutMin=[]  SumDOutMax=[]  DifferentiatorOutMin=[]  DifferentiatorOutMax=[]  FilterDiffOutCoefMin=[]  FilterDiffOutCoefMax=[]  ReciprocalOutMin=[]  ReciprocalOutMax=[]  SumDenOutMin=[]  SumDenOutMax=[]  SumNumOutMin=[]  SumNumOutMax=[]  DivideOutMin=[]  DivideOutMax=[]  UdiffTsProdOutMin=[]  UdiffTsProdOutMax=[]  NTsProdOutMin=[]  NTsProdOutMax=[]  UintegralTsProdOutMin=[]  UintegralTsProdOutMax=[]  UngainTsProdOutMin=[]  UngainTsProdOutMax=[]  ClampingZeroOutDataTypeStr=Inherit: Inherit via back propagation  ClampingZeroOutMin=[]  ClampingZeroOutMax=[]  FilterDenConstantOutDataTypeStr=Inherit: Inherit via back propagation  FilterDenConstantOutMin=[]  FilterDenConstantOutMax=[]  PCopyOutDataTypeStr=Inherit: Inherit via back propagation  PCopyOutMin=[]  PCopyOutMax=[]  NCopyOutDataTypeStr=Inherit: Inherit via back propagation  NCopyOutMin=[]  NCopyOutMax=[]  IntegratorContinuousStateAttributes=''  IntegratorStateMustResolveToSignalObject=off  IntegratorRTWStateStorageClass=Auto  FilterContinuousStateAttributes=''  FilterStateMustResolveToSignalObject=off  FilterRTWStateStorageClass=Auto  ParallelPVariant=InternalParameters  IdealPVariant=Disabled  IVariant=InternalParameters  DVariant=InternalParameters  IntegratorVariant=Continuous  SatVariant=Disabled  AWVariant=Passthrough  PCopyVariant=Disabled  TRVariant=Disabled  FdbkBlocksVariant=Forward  IdealPFdbkVariant=Disabled  SatFdbkVariant=Disabled  DerivativeFilterVariant=ContFilter  NVariant=InternalParameters  NCopyVariant=Disabled  FilterICVariant=InternalICsFilter  IntegratorICVariant=InternalICs  ExternalResetVariant=Disabled  TRSumVariant=Passthrough  SumFdbkVariant=Disabled  SumVariant=Sum_PID  TsampFilterVariant=InternalTs  TsampNgainVariant=Passthrough  TsampIntegralVariant=Disabled_SignalSpec  ExternalSaturationOutDataTypeStr=Inherit: Same as second input  DerivativeSourceVariant=ErrorSignal  PreIntVariant=InternalPreInt
  Product2 : Product  RndMeth=Zero
  Product3 : Product
  Product4 : Product  Inputs=*/  RndMeth=Zero
  Saturation_Dynamic : simulink/Discontinuities/Saturation Dynamic  OutMin=[]  OutMax=[]  OutDataTypeStr=Inherit: Same as second input  OutDataType=fixdt(1, 16)  OutScaling=2^-10  DoSatur=off
  Sum2 : Sum  Inputs=+-|
  Sum3 : Sum  Inputs=|++
  mot_propel_plant_init_eff_map : Subsystem  mask{x=mot4.propel.plant.init.CP_CT_map(:,1)/60, map=mot4.propel.plant.init.CP_CT_map(:,4)}
  mot_ctrl_trs_trq_simu : Outport  VectorParamsAs1DForOutWhenUnconnected=off
  mot_ctrl_ratedpwr_simu : Outport  Port=2
  wires:
  Product2/1 -> Product3/1
  mot_propel_plant_init_eff_map/1(output) -> Product3/2
  Constant/1 -> mot_ctrl_ratedpwr_simu/1, Product2/1  "mot_ctrl_ratedpwr_simu"
  Constant3/1 -> Saturation_Dynamic/3
  tc_plant_spd_in_simu/1 -> Gain/1
  Saturation_Dynamic/1 -> Determine_Required_Motor_RPS/3(P), Product4/1
  Product3/1 -> Saturation_Dynamic/2
  Gain/1 -> Sum2/2  "actual"
  Product4/1 -> Sum3/1  "required"
  PID Controller/1 -> Sum3/2
  Sum3/1 -> mot_ctrl_trs_trq_simu/1  "mot_ctrl_trs_trq_simu"
  1\2pi1/1 -> Product4/2
  Sum2/1 -> PID Controller/1
  apc_ctrl_dt_simu/1 -> Product2/2
  ess_ctrl_pwr_max_pro_simu/1 -> Saturation_Dynamic/1
  propel_plant_speed_simu/1 -> Gain1/1
  Determine_Required_Motor_RPS/1(RPS_req) -> Sum2/1, 1\2pi1/1
  Constant8/1 -> Determine_Required_Motor_RPS/1(Prop_D)
  env_plant_density_simu/1 -> Determine_Required_Motor_RPS/2(rho)
  Constant2/1 -> Determine_Required_Motor_RPS/4(CPpoly)
  Gain1/1 -> mot_propel_plant_init_eff_map/1(input x)

== system AeroPropRefFranc/Propulsion and Aerodynamic Forces and Moments/S-Function/Battery Model/powerplant/mot4/ctrl/dmd/parameter_out ==
  inport-mot4_ctrl_trs_trq_simu : Inport
  inport-mot4_ctrl_ratedpwr_simu : Inport  Port=2
  Ground_1 : Ground
  Toworkspace-mot4_ctrl_ratedpwr_simu : ToWorkspace  VariableName=mot4_ctrl_ratedpwr_simu  SampleTime=pxf_diagram_options.workspace_sample_time
      settings: Decimation=pxf_diagram_options.decimation
  Toworkspace-mot4_ctrl_trs_trq_simu : ToWorkspace  VariableName=mot4_ctrl_trs_trq_simu  SampleTime=pxf_diagram_options.workspace_sample_time
      settings: Decimation=pxf_diagram_options.decimation
  create_system_info_bus : BusCreator  Inputs=1
  outport-system_info_bus : Outport
  outport-dmd_bus : Outport  Port=2
  wires:
  Ground_1/1 -> outport-dmd_bus/1
  inport-mot4_ctrl_ratedpwr_simu/1 -> Toworkspace-mot4_ctrl_ratedpwr_simu/1
  inport-mot4_ctrl_trs_trq_simu/1 -> Toworkspace-mot4_ctrl_trs_trq_simu/1, create_system_info_bus/1  "mot4_ctrl_trs_trq_simu"
  create_system_info_bus/1 -> outport-system_info_bus/1

== system AeroPropRefFranc/Propulsion and Aerodynamic Forces and Moments/S-Function/Battery Model/powerplant/mot4/ctrl/dmd/parameter_selection ==
  inport-main_info_bus-1 : Inport
  select_main_info_bus : BusSelector  OutputSignals=apc_info_bus.apc_ctrl_dt4_simu,env_info_bus.env_plant_density_simu,apa_info_bus.powerplant_info_bus.ess.ctrl.ess_ctrl_pwr_max_pro_simu,apa_info_bus.powerplant_info_bus.propel4.propel4_plant_speed_simu,apa_info_bus.powerplant_info_bus.tc4.tc4_plant_spd_in_simu
  outport-apc_ctrl_dt4_simu-1 : Outport
  outport-env_plant_density_simu-2 : Outport  Port=2
  outport-ess_ctrl_pwr_max_pro_simu-3 : Outport  Port=3
  outport-propel4_plant_speed_simu-4 : Outport  Port=4
  outport-tc4_plant_spd_in_simu-5 : Outport  Port=5
  wires:
  select_main_info_bus/5 -> outport-tc4_plant_spd_in_simu-5/1  "<tc4_plant_spd_in_simu>"
  select_main_info_bus/4 -> outport-propel4_plant_speed_simu-4/1  "<propel4_plant_speed_simu>"
  select_main_info_bus/3 -> outport-ess_ctrl_pwr_max_pro_simu-3/1  "<ess_ctrl_pwr_max_pro_simu>"
  select_main_info_bus/2 -> outport-env_plant_density_simu-2/1  "<env_plant_density_simu>"
  select_main_info_bus/1 -> outport-apc_ctrl_dt4_simu-1/1  "<apc_ctrl_dt4_simu>"
  inport-main_info_bus-1/1 -> select_main_info_bus/1

== system AeroPropRefFranc/Propulsion and Aerodynamic Forces and Moments/S-Function/Battery Model/powerplant/mot4/plant/mot4_plant_map_Pelec_funTW_volt_in/electric machine filter ==
  trq : Inport
  Interval Test : simulink/Logic and Bit Operations/Interval Test  IntervalClosedRight=on  uplimit=0.02  IntervalClosedLeft=on  lowlimit=-0.02  OutDataTypeStr=boolean
  Switch : Switch  Threshold=0.5  SaturateOnIntegerOverflow=off  InputSameDT=off
  electric machine time response : TransferFcn  Denominator=[mot4.plant.init.time_response 1]
  filtered : Outport
  wires:
  electric machine time response/1 -> Switch/3
  Interval Test/1 -> Switch/2
  trq/1 -> Switch/1, Interval Test/1, electric machine time response/1
  Switch/1 -> filtered/1

== system AeroPropRefFranc/Propulsion and Aerodynamic Forces and Moments/S-Function/Battery Model/powerplant/mot4/plant/mot4_plant_map_Pelec_funTW_volt_in/max torque  ==
  cmd : Inport
  speed : Inport  Port=2
  torque : Inport  Port=3
  Abs : Abs
  Cont trq max - Prop : Subsystem  mask{x=mot4.plant.init.trq_pos_cont.idx1_spd, map=mot4.plant.init.trq_pos_cont.map}
      mask Display: image(imread('map1D.jpg','jpeg'))
  Cont trq max - Regen : Subsystem  mask{x=mot4.plant.init.trq_neg_cont.idx1_spd, map=mot4.plant.init.trq_neg_cont.map}
      mask Display: image(imread('map1D.jpg','jpeg'))
  Heat index : Subsystem
  Memory : Memory
  Peak trq max - Prop : Subsystem  mask{x=mot4.plant.init.trq_pos_max.idx1_spd, map=mot4.plant.init.trq_pos_max.map}
      mask Display: image(imread('map1D.jpg','jpeg'))
  Peak trq max - Regen : Subsystem  mask{x=mot4.plant.init.trq_neg_max.idx1_spd, map=mot4.plant.init.trq_neg_max.map}
      mask Display: image(imread('map1D.jpg','jpeg'))
  Product2 : Product  InputSameDT=on  SaturateOnIntegerOverflow=on  OutDataTypeStr=Inherit: Same as first input
  Product3 : Product  InputSameDT=on  SaturateOnIntegerOverflow=on  OutDataTypeStr=Inherit: Same as first input
  Product5 : Product  InputSameDT=on  SaturateOnIntegerOverflow=on  OutDataTypeStr=Inherit: Same as first input
  Sign : Signum
  Sum : Sum  InputSameDT=on  SaturateOnIntegerOverflow=on  OutDataTypeStr=Inherit: Same as first input
  Sum1 : Sum  Inputs=-+  InputSameDT=on  SaturateOnIntegerOverflow=on  OutDataTypeStr=Inherit: Same as first input
  Switch : Switch  InputSameDT=off
  Switch1 : Switch  InputSameDT=off
  cst : Constant
  max torque : Outport
  heat index : Outport  Port=2
  wires:
  Heat index/1(Heat index) -> heat index/1, Sum1/1, Product2/2
  cst/1 -> Sum1/2
  Product3/1 -> Sum/2
  Sum1/1 -> Product3/1
  Product2/1 -> Sum/1
  Switch1/1 -> Product3/2
  Switch/1 -> Heat index/1(cont torque), Product2/1
  Peak trq max - Regen/1(output) -> Switch1/3
  Peak trq max - Prop/1(output) -> Switch1/1
  Cont trq max - Regen/1(output) -> Switch/3
  Cont trq max - Prop/1(output) -> Switch/1
  speed/1 -> Memory/1
  cmd/1 -> Switch/2, Switch1/2
  torque/1 -> Heat index/2(torque)
  Abs/1 -> Product5/2
  Sum/1 -> Abs/1, Sign/1
  Product5/1 -> max torque/1
  Sign/1 -> Product5/1
  Memory/1 -> Peak trq max - Prop/1(input x), Peak trq max - Regen/1(input x), Cont trq max - Regen/1(input x), Cont trq max - Prop/1(input x)
